simulink model "Misc_operators"  (R2013b)
settings: Solver=ode45  StartTime=0.0  StopTime=10.0  RelTol=1e-3
undefined symbols (not defined in the file): epsilon
settings Model: Creator=rskjetne  LastModifiedBy=rskjetne

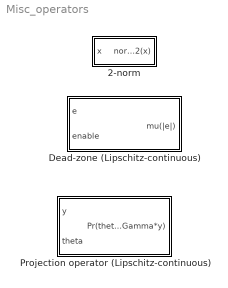
== system Misc_operators ==
  2-norm : Subsystem
  Dead-zone (Lipschitz-continuous) : Subsystem  mask{e0=0.1, delta=0.5}
      mask prompts: e0 "e0: 0 < e0"; delta "delta: 0 < delta < 1"
  Projection operator (Lipschitz-continuous) : Subsystem  mask{e0=0.5, theta_max=10, Gamma=eye(1)}
      mask prompts: e0 "epsilon: eps > 0"; theta_max "Max limit: theta_max"; Gamma "Gain matrix: Gamma"

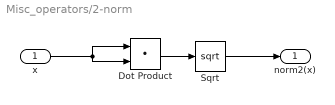
== system Misc_operators/2-norm ==
  x : Inport
  Dot Product : DotProduct  InputSameDT=on  OutDataTypeStr=Inherit: Inherit via internal rule
  Sqrt : Sqrt  SaturateOnIntegerOverflow=on
  norm2(x) : Outport
  wires:
  x/1 -> Dot Product/2, Dot Product/1
  Sqrt/1 -> norm2(x)/1
  Dot Product/1 -> Sqrt/1

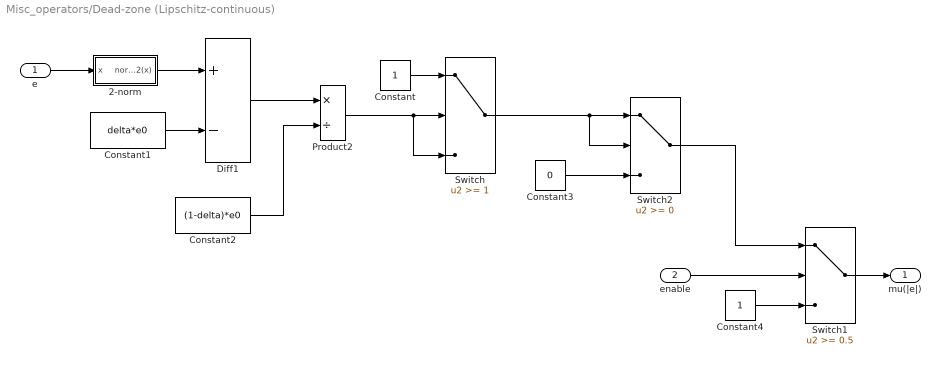
== system Misc_operators/Dead-zone (Lipschitz-continuous) ==
  e : Inport
  enable : Inport  Port=2
  2-norm : Subsystem
  Constant : Constant
  Constant1 : Constant  Value=delta*e0
  Constant2 : Constant  Value=(1-delta)*e0
  Constant3 : Constant  Value=0
  Constant4 : Constant
  Diff1 : Sum  Inputs=+-  InputSameDT=on  OutDataTypeStr=Inherit: Same as first input
  Product2 : Product  Inputs=*/
  Switch : Switch  Threshold=1  ZeroCross=off  InputSameDT=on
  Switch1 : Switch  Threshold=0.5  ZeroCross=off  InputSameDT=on
  Switch2 : Switch  ZeroCross=off  InputSameDT=on
  mu(|e|) : Outport
  wires:
  Constant1/1 -> Diff1/2
  Diff1/1 -> Product2/1
  Constant2/1 -> Product2/2
  Product2/1 -> Switch/3, Switch/2
  Constant/1 -> Switch/1
  Switch/1 -> Switch2/1, Switch2/2
  Constant3/1 -> Switch2/3
  e/1 -> 2-norm/1(x)
  2-norm/1(norm2(x)) -> Diff1/1
  enable/1 -> Switch1/2
  Switch2/1 -> Switch1/1
  Switch1/1 -> mu(|e|)/1
  Constant4/1 -> Switch1/3

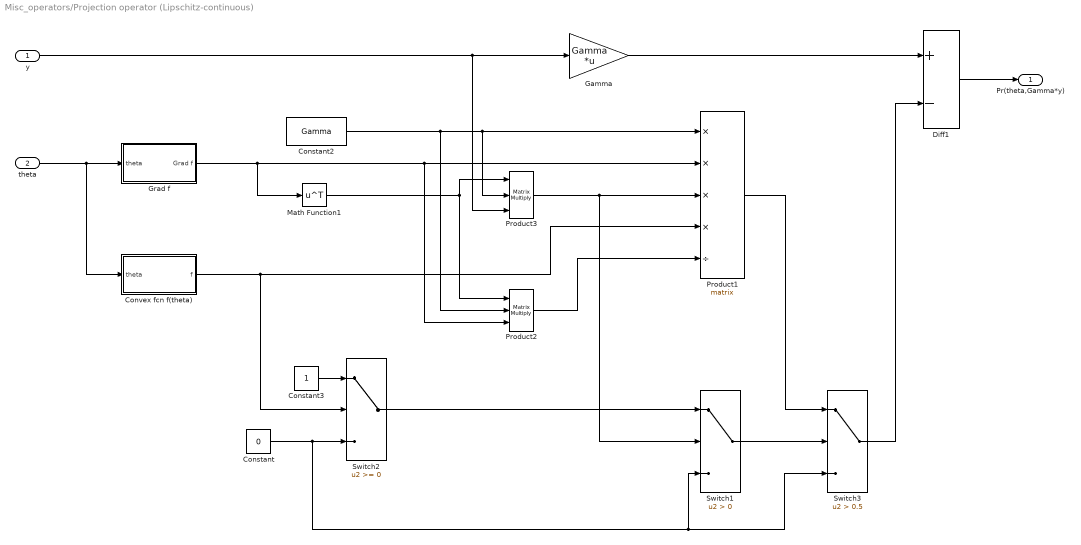
== system Misc_operators/Projection operator (Lipschitz-continuous) ==
  y : Inport
  theta : Inport  Port=2
  Constant : Constant  Value=0
  Constant2 : Constant  Value=Gamma
  Constant3 : Constant
  Convex fcn f(theta) : Subsystem
  Diff1 : Sum  Inputs=+-  InputSameDT=on  OutDataTypeStr=Inherit: Same as first input
  Gamma : Gain  Gain=Gamma  Multiplication=Matrix(K*u)  SaturateOnIntegerOverflow=on  OutDataTypeStr=Inherit: Same as input  ParamDataTypeStr=Inherit: Same as input
  Grad f : Subsystem
  Math Function1 : Math  Operator=transpose  SaturateOnIntegerOverflow=on
  Product1 : Product  Inputs=****/  Multiplication=Matrix(*)
  Product2 : Product  Inputs=***  Multiplication=Matrix(*)
  Product3 : Product  Inputs=***  Multiplication=Matrix(*)
  Switch1 : Switch  Criteria=u2 > Threshold  ZeroCross=off  InputSameDT=on
  Switch2 : Switch  ZeroCross=off  InputSameDT=on
  Switch3 : Switch  Criteria=u2 > Threshold  Threshold=0.5  ZeroCross=off  InputSameDT=on
  Pr(theta,Gamma*y) : Outport
  wires:
  Diff1/1 -> Pr(theta,Gamma*y)/1
  Constant/1 -> Switch3/3, Switch1/3, Switch2/3
  Switch2/1 -> Switch1/1
  Constant3/1 -> Switch2/1
  Product3/1 -> Product1/3, Switch1/2
  Product2/1 -> Product1/5
  Grad f/1(Grad f) -> Product1/2, Product2/3, Math Function1/1
  Convex fcn f(theta)/1(f) -> Product1/4, Switch2/2
  Math Function1/1 -> Product3/1, Product2/1
  Constant2/1 -> Product1/1, Product3/2, Product2/2
  Gamma/1 -> Diff1/1
  y/1 -> Gamma/1, Product3/3
  theta/1 -> Grad f/1(theta), Convex fcn f(theta)/1(theta)
  Switch1/1 -> Switch3/2
  Product1/1 -> Switch3/1
  Switch3/1 -> Diff1/2

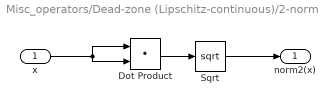
== system Misc_operators/Dead-zone (Lipschitz-continuous)/2-norm ==
  x : Inport
  Dot Product : DotProduct  InputSameDT=on  OutDataTypeStr=Inherit: Inherit via internal rule
  Sqrt : Sqrt  SaturateOnIntegerOverflow=on
  norm2(x) : Outport
  wires:
  x/1 -> Dot Product/2, Dot Product/1
  Sqrt/1 -> norm2(x)/1
  Dot Product/1 -> Sqrt/1

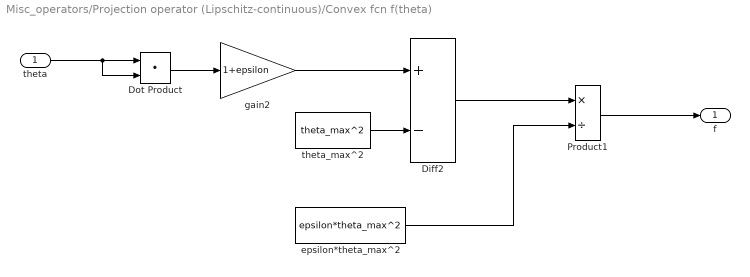
== system Misc_operators/Projection operator (Lipschitz-continuous)/Convex fcn f(theta) ==
  theta : Inport
  Diff2 : Sum  Inputs=+-  InputSameDT=on  OutDataTypeStr=Inherit: Same as first input
  Dot Product : DotProduct  InputSameDT=on  OutDataTypeStr=Inherit: Inherit via internal rule
  Product1 : Product  Inputs=*/
  epsilon*theta_max^2 : Constant  Value=epsilon*theta_max^2
  gain2 : Gain  Gain=1+epsilon  SaturateOnIntegerOverflow=on  OutDataTypeStr=Inherit: Same as input  ParamDataTypeStr=Inherit: Same as input
  theta_max^2 : Constant  Value=theta_max^2
  f : Outport
  wires:
  Diff2/1 -> Product1/1
  epsilon*theta_max^2/1 -> Product1/2
  Product1/1 -> f/1
  theta_max^2/1 -> Diff2/2
  theta/1 -> Dot Product/1, Dot Product/2
  gain2/1 -> Diff2/1
  Dot Product/1 -> gain2/1

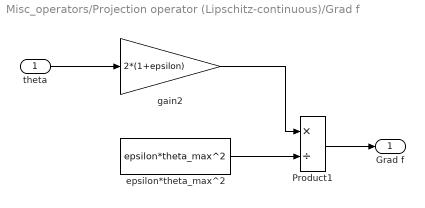
== system Misc_operators/Projection operator (Lipschitz-continuous)/Grad f ==
  theta : Inport
  Product1 : Product  Inputs=*/
  epsilon*theta_max^2 : Constant  Value=epsilon*theta_max^2
  gain2 : Gain  Gain=2*(1+epsilon)  SaturateOnIntegerOverflow=on  OutDataTypeStr=Inherit: Same as input  ParamDataTypeStr=Inherit: Same as input
  Grad f : Outport
  wires:
  theta/1 -> gain2/1
  gain2/1 -> Product1/1
  Product1/1 -> Grad f/1
  epsilon*theta_max^2/1 -> Product1/2
